simulink model "Gercek_Model_Non_Linear_Ters_Sarkac"  (R2022a)
settings: Solver=ode4  StartTime=0.0  StopTime=10.0  FixedStep=1/1000  RelTol=1e-3
InitFcn:
  | Sarkac_Parametrelerini_Yukle
values from neighbouring files (symbols this model uses):
  b = 0.1    [Sarkac_Parametrelerini_Yukle.m]
  Baslangic_Degerleri = [0,0,pi,0]    [Sarkac_Parametrelerini_Yukle.m]
  g = 9.8    [Sarkac_Parametrelerini_Yukle.m]
  I = 0.006    [Sarkac_Parametrelerini_Yukle.m]
  l = 0.3    [Sarkac_Parametrelerini_Yukle.m]
  M = 0.5    [Sarkac_Parametrelerini_Yukle.m]
  m = 0.2    [Sarkac_Parametrelerini_Yukle.m]
undefined symbols (not defined in the file or in its folder): sigbuilder_block
libraries: vrlib x1
settings Model: Creator=Fatabi  LastModifiedBy=Fatabi
settings SolverCC: AlgebraicLoopSolver=TrustRegion
settings DebuggingCC: UnconnectedInputMsg=warning  UnconnectedOutputMsg=warning  UnconnectedLineMsg=warning  SFMachineParentedDataDiag=warning

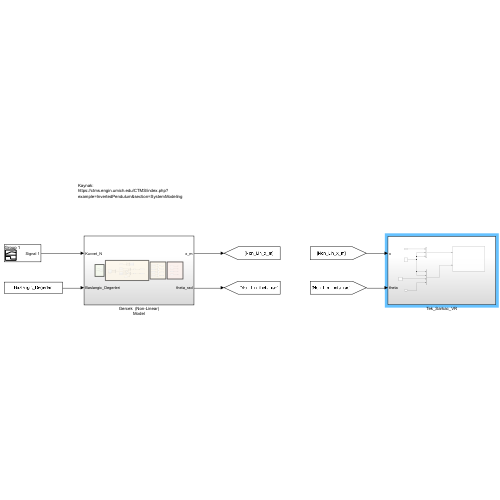
[thumbnail: Simulink's stored preview of the top-level diagram]
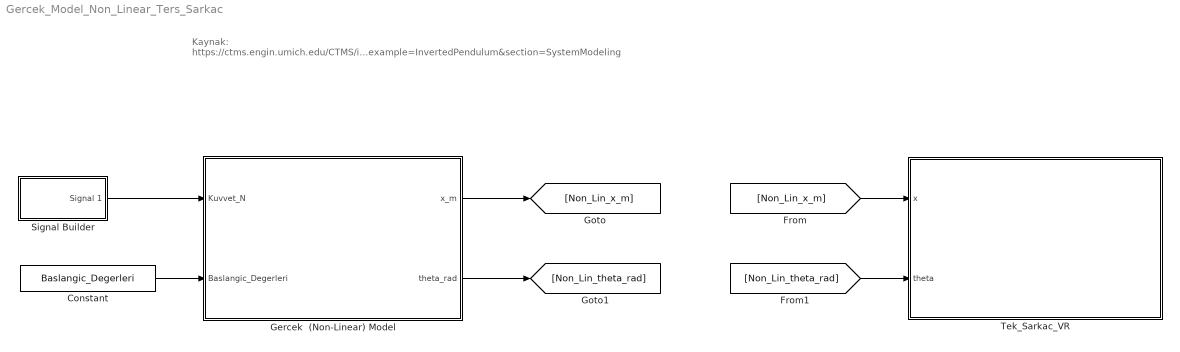
== system Gercek_Model_Non_Linear_Ters_Sarkac ==
  note: Kaynak:
      | https://ctms.engin.umich.edu/CTMS/index.php?example=InvertedPendulum&section=SystemModeling
  Constant : Constant  Value=Baslangic_Degerleri
  Gercek  (Non-Linear) Model : Subsystem
  Signal Builder : Subsystem  Tag=STV Subsys  LoadFcn=sigbuilder_block('load');  StartFcn=sigbuilder_block('start');  StopFcn=sigbuilder_block('stop');  ClipboardFcn=sigbuilder_block('clipboard');  mask(Sigbuilder block){tuvar=[0:10]}
      mask help: Simulink:masks:SigbuilderBlock_MD
      mask init:
      | if ~strcmp(get_param(bdroot(gcbh),'SimulationStatus'),'stopped') tuvar = sigbuilder_block('maskInit'); end
      settings: CopyFcn=sigbuilder_block('copy');  DeleteFcn=sigbuilder_block('delete');  ModelCloseFcn=sigbuilder_block('modelClose');  PreSaveFcn=sigbuilder_block('preSave');  PauseFcn=sigbuilder_block('pause');  ContinueFcn=sigbuilder_block('continue');  NameChangeFcn=sigbuilder_block('namechange');  OpenFcn=sigbuilder_block('open',[338.25 225.75 550.5 399.75 ]);  CloseFcn=sigbuilder_block('close');
      mask Display: plot(0, 0, 100, 100,[2, 2, 32, 32, 2], [68, 8, 8, 68, 68],[32, 2], [38, 38], [32, 19, 2],[53, 60, 44], [32, 17, 17, 2],[16, 16, 31, 31]);txt = getActiveGroup(gcbh);text(2, 100, txt,'verticalAlignment', 'top');
  "Tek_Sarkac_VR " : Subsystem
  wires:
  Signal Builder/1(Signal 1) -> Gercek  (Non-Linear) Model/1(Kuvvet_N)
  Constant/1 -> Gercek  (Non-Linear) Model/2(Baslangic_Degerleri)
  Gercek  (Non-Linear) Model/1(x_m) -> [Non_Lin_x_m]
  Gercek  (Non-Linear) Model/2(theta_rad) -> [Non_Lin_theta_rad]
  [Non_Lin_x_m] -> "Tek_Sarkac_VR "/1(x)
  [Non_Lin_theta_rad] -> "Tek_Sarkac_VR "/2("theta ")

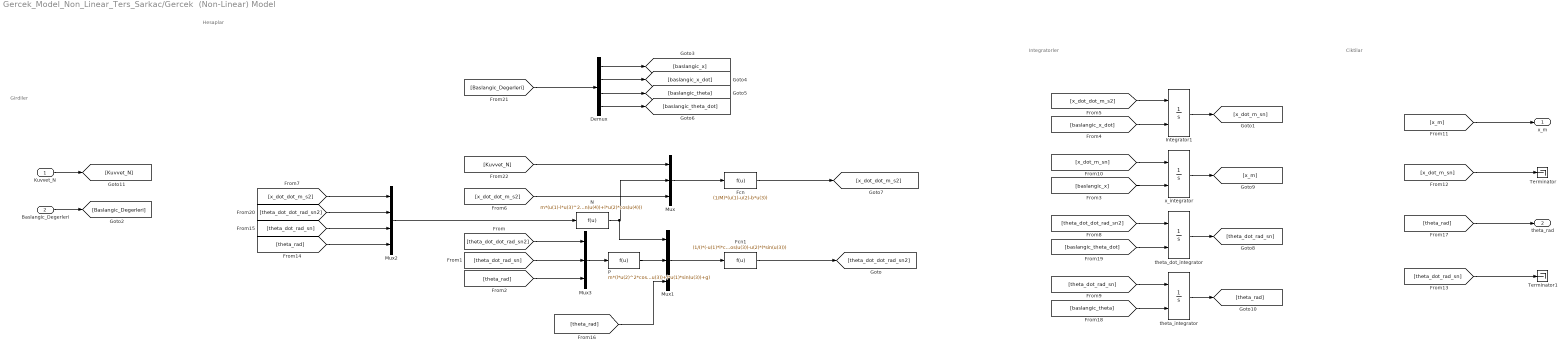
== system Gercek_Model_Non_Linear_Ters_Sarkac/Gercek  (Non-Linear) Model ==
  note: Integratorler
  note: Girdiler
  note: Ciktilar
  note: Hesaplar
  Kuvvet_N : Inport
  Baslangic_Degerleri : Inport  Port=2
  Demux : Demux
  Fcn : Fcn  Expr=(1/M)*(u(1)-u(2)-b*u(3))
  Fcn1 : Fcn  Expr=(1/I)*(-u(1)*l*cos(u(3))-u(2)*l*sin(u(3)))
  Integrator1 : Integrator  InitialConditionSource=external  ContinuousStateAttributes='x_dot_m_sn'
  Mux : Mux  Inputs=3
  Mux1 : Mux  Inputs=3
  Mux2 : Mux
  Mux3 : Mux  Inputs=3
  N : Fcn  Expr=m*(u(1)-l*u(3)^2*sin(u(4))+l*u(2)*cos(u(4)))
  P : Fcn  Expr=m*(l*u(2)^2*cos(u(3))+l*u(1)*sin(u(3))+g)
  Terminator : Terminator
  Terminator1 : Terminator
  theta_dot_integrator : Integrator  InitialConditionSource=external  ContinuousStateAttributes='theta_dot_rad_sn'
  theta_integrator : Integrator  InitialConditionSource=external  InitialCondition=pi-0.1  ContinuousStateAttributes='theta_rad'
  x_integrator : Integrator  InitialConditionSource=external  ContinuousStateAttributes='x_m'
  x_m : Outport
  theta_rad : Outport  Port=2
  wires:
  [x_dot_dot_m_s2] -> Mux/3
  Fcn/1 -> [x_dot_dot_m_s2]
  [Kuvvet_N] -> Mux/1
  N/1 -> Mux1/1, Mux/2
  Mux/1 -> Fcn/1
  Fcn1/1 -> [theta_dot_dot_rad_sn2]
  Mux1/1 -> Fcn1/1
  P/1 -> Mux1/2
  Mux2/1 -> N/1
  [theta_dot_dot_rad_sn2] -> Mux3/1
  [theta_dot_rad_sn] -> Mux3/2
  [theta_rad] -> Mux3/3
  Mux3/1 -> P/1
  [Baslangic_Degerleri] -> Demux/1
  Demux/1 -> [baslangic_x]
  Demux/2 -> [baslangic_x_dot]
  Demux/3 -> [baslangic_theta]
  Demux/4 -> [baslangic_theta_dot]
  [baslangic_x] -> x_integrator/2
  x_integrator/1 -> [x_m]
  [baslangic_x_dot] -> Integrator1/2
  [x_dot_dot_m_s2] -> Integrator1/1
  Integrator1/1 -> [x_dot_m_sn]
  [x_dot_dot_m_s2] -> Mux2/1
  [theta_dot_dot_rad_sn2] -> theta_dot_integrator/1
  theta_dot_integrator/1 -> [theta_dot_rad_sn]
  [x_dot_m_sn] -> x_integrator/1
  [x_m] -> x_m/1
  [x_dot_m_sn] -> Terminator/1
  [theta_dot_rad_sn] -> theta_integrator/1
  theta_integrator/1 -> [theta_rad]
  [theta_rad] -> Mux2/4
  [theta_dot_rad_sn] -> Mux2/3
  [theta_rad] -> Mux1/3
  [theta_rad] -> theta_rad/1
  [baslangic_theta] -> theta_integrator/2
  [baslangic_theta_dot] -> theta_dot_integrator/2
  [theta_dot_dot_rad_sn2] -> Mux2/2
  Baslangic_Degerleri/1 -> [Baslangic_Degerleri]
  Kuvvet_N/1 -> [Kuvvet_N]
  [theta_dot_rad_sn] -> Terminator1/1

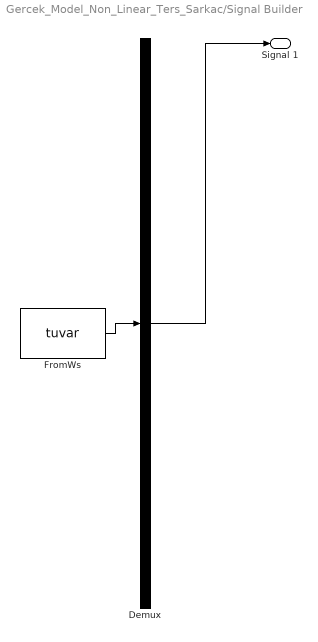
== system Gercek_Model_Non_Linear_Ters_Sarkac/Signal Builder ==
  Demux : Demux  Tag=STV Demux  Outputs=1
      settings: DisplayOption=none
  FromWs : FromWorkspace  Tag=STV FromWs  VariableName=tuvar
      SigBuilderData=|
      | common.afterFinalStr = 'Extrapolate'
      | common.sampleTime = 0
      | dataSet.timeRange = [0 10]
      | dataSet.name = 'Group 1'
      | sbobj.Groups.Name = 'Group 1'
      | sbobj.Groups.Signals.Name = 'Signal 1'
      | sbobj.Groups.Signals.XData = [0 1 1 1.5 1.5 10]
      | sbobj.Groups.Signals.YData = [0 0 1 1 0 0]
  Signal 1 : Outport  Tag=STV Outport
  wires:
  Demux/1 -> Signal 1/1
  FromWs/1 -> Demux/1

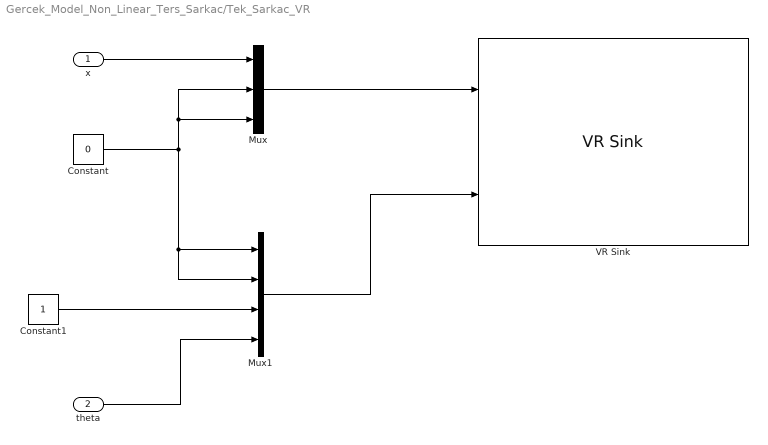
== system Gercek_Model_Non_Linear_Ters_Sarkac/Tek_Sarkac_VR  ==
  x : Inport
  "theta " : Inport  Port=2
  Constant : Constant  Value=0
  Constant1 : Constant
  Mux : Mux  Inputs=3
  Mux1 : Mux
  VR Sink : vrlib/VR Sink  InstantiateOnLoad=on  SampleTime=0.02  ViewEnable=on  RemoteChange=off  RemoteView=off  FieldsWritten=Kutu.translation.3.1.1.double#Mentese1.rotation.4.1.1.double  WorldFileName=sarkac.wrl  AutoView=off  VideoDimensions=[]  AllowVariableSize=off
  wires:
  x/1 -> Mux/1
  Constant/1 -> Mux/3, Mux/2, Mux1/2, Mux1/1
  "theta "/1 -> Mux1/4
  Constant1/1 -> Mux1/3
  Mux/1 -> VR Sink/1
  Mux1/1 -> VR Sink/2
